simulink model "TRAMI_DCT_AT"  (R2018b)
settings: Solver=FixedStepDiscrete  StartTime=0.0  StopTime=88  FixedStep=10e-3  RelTol=1e-3  EnableMultiTasking=on
undefined symbols (not defined in the file): CONST_AP_GEAR_SUB_NEWTRAL, CONST_AP_IDLE_SPEED_CONT, CONST_AP_LOAD_SFT, CONST_AP_LOAD_SFT_HYS, CONST_CAR_WEIGHT, CONST_CL_NUM, CONST_F_DOWN_SYNCHRO, CONST_F_SYNCHRO, CONST_F_UP_SYNCHRO, CONST_FGR, CONST_I_FlYWHEEL, CONST_INATIA_CLANK, CONST_R_SHIFT_END_CD, CONST_R_SHIFT_END_EG, CONST_R_SHIFT_END_TD, CONST_R_SHIFT_END_UP, CONST_R_SYNCHRO_ENGAGE, CONST_R_TIRE, CONST_RATIO_TQ_REDUCTION, CONST_SKIP_SHIFT_MAX, CONST_SYN_NUM, CONST_T_SFT_END_EN, CONST_T_SFT_END_JUDGE, CONST_T_SFT_END_MAX, CONST_T_SFT_END_MIN, CONST_T_SHIFT_WAIT, CONST_T_TQ_PHASE_CD, CONST_T_TQ_PHASE_ND, CONST_T_TQ_PHASE_NR, CONST_T_TQ_PHASE_TD, CONST_T_TQ_PHASE_UP, CONST_TQ_CREEP_CONT, CONST_TQ_ENGAGE_CL_MARGIN, CONST_TQ_ENGAGE_CL_MIN, CONST_TQ_INATIA_TD_SHIFT, CONST_TQ_LOAD_SFT, CONST_TQ_LOAD_SFT_HYS, CONST_TQ_ND_ENGAGE, CONST_TQ_NR_ENGAGE, CONST_TQ_TQPHASE_MIN, CONST_V_IDLE_SPEED_CONT, Eng, FALSE, GrNP, GrRev, LoopTime, MAT_CL_ENGAGE, MAT_CL_SHARE_RATE, MAT_I_ACTUATOR, MAT_SYNCHRO_COM, MAT_T_GEAR_SUB_NEWTRAL, MAT_TRANS_MGR, MaxCL, Nm, PI, Shift_CD, Shift_ND, Shift_NR, Shift_TD, Shift_Up ... (+168)
libraries: simulink x26
(part 6 of 6)

== system TRAMI_DCT_AT/TCU_Main/StartingDeviceControl/StartingDeviceControl/TCU_Slip_Control/Table_search_3D_G10 ==
  X : Inport  OutDataTypeStr=single
  Y : Inport  Port=2  OutDataTypeStr=single
  1-D Lookup Table1 : Lookup_n-D  NumberOfTableDimensions=1  BreakpointsForDimension1=axis_x  Table=tbl_x  ExtrapMethod=Clip  InternalRulePriority=Speed  OutDataTypeStr=single  RndMeth=Simplest  InputSameDT=on
  1-D Lookup Table2 : Lookup_n-D  NumberOfTableDimensions=1  BreakpointsForDimension1=axis_y  Table=tbl_y  ExtrapMethod=Clip  InternalRulePriority=Speed  OutDataTypeStr=single  RndMeth=Simplest  InputSameDT=on
  2-D Lookup Table : Lookup_n-D  BreakpointsForDimension1=tbl_y  BreakpointsForDimension2=tbl_x  Table=map  ExtrapMethod=Clip  InternalRulePriority=Speed  OutDataTypeStr=single  RndMeth=Simplest  InputSameDT=on
  out : Outport  OutDataTypeStr=single
  wires:
  1-D Lookup Table1/1 -> 2-D Lookup Table/2  "x_nrm"
  1-D Lookup Table2/1 -> 2-D Lookup Table/1  "y_nrm"
  Y/1 -> 1-D Lookup Table2/1  "data_y"
  X/1 -> 1-D Lookup Table1/1  "data_x"
  2-D Lookup Table/1 -> out/1

== system TRAMI_DCT_AT/TCU_Main/StartingDeviceControl/StartingDeviceControl/TCU_Slip_Control/Table_search_3D_G2 ==
  X : Inport  OutDataTypeStr=single
  Y : Inport  Port=2  OutDataTypeStr=single
  1-D Lookup Table1 : Lookup_n-D  NumberOfTableDimensions=1  BreakpointsForDimension1=axis_x  Table=tbl_x  ExtrapMethod=Clip  InternalRulePriority=Speed  OutDataTypeStr=single  RndMeth=Simplest  InputSameDT=on
  1-D Lookup Table2 : Lookup_n-D  NumberOfTableDimensions=1  BreakpointsForDimension1=axis_y  Table=tbl_y  ExtrapMethod=Clip  InternalRulePriority=Speed  OutDataTypeStr=single  RndMeth=Simplest  InputSameDT=on
  2-D Lookup Table : Lookup_n-D  BreakpointsForDimension1=tbl_y  BreakpointsForDimension2=tbl_x  Table=map  ExtrapMethod=Clip  InternalRulePriority=Speed  OutDataTypeStr=single  RndMeth=Simplest  InputSameDT=on
  out : Outport  OutDataTypeStr=single
  wires:
  1-D Lookup Table1/1 -> 2-D Lookup Table/2  "x_nrm"
  1-D Lookup Table2/1 -> 2-D Lookup Table/1  "y_nrm"
  Y/1 -> 1-D Lookup Table2/1  "data_y"
  X/1 -> 1-D Lookup Table1/1  "data_x"
  2-D Lookup Table/1 -> out/1

== system TRAMI_DCT_AT/TCU_Main/StartingDeviceControl/StartingDeviceControl/TCU_Slip_Control/Table_search_3D_G3 ==
  X : Inport  OutDataTypeStr=single
  Y : Inport  Port=2  OutDataTypeStr=single
  1-D Lookup Table1 : Lookup_n-D  NumberOfTableDimensions=1  BreakpointsForDimension1=axis_x  Table=tbl_x  ExtrapMethod=Clip  InternalRulePriority=Speed  OutDataTypeStr=single  RndMeth=Simplest  InputSameDT=on
  1-D Lookup Table2 : Lookup_n-D  NumberOfTableDimensions=1  BreakpointsForDimension1=axis_y  Table=tbl_y  ExtrapMethod=Clip  InternalRulePriority=Speed  OutDataTypeStr=single  RndMeth=Simplest  InputSameDT=on
  2-D Lookup Table : Lookup_n-D  BreakpointsForDimension1=tbl_y  BreakpointsForDimension2=tbl_x  Table=map  ExtrapMethod=Clip  InternalRulePriority=Speed  OutDataTypeStr=single  RndMeth=Simplest  InputSameDT=on
  out : Outport  OutDataTypeStr=single
  wires:
  2-D Lookup Table/1 -> out/1
  X/1 -> 1-D Lookup Table1/1  "data_x"
  Y/1 -> 1-D Lookup Table2/1  "data_y"
  1-D Lookup Table2/1 -> 2-D Lookup Table/1  "y_nrm"
  1-D Lookup Table1/1 -> 2-D Lookup Table/2  "x_nrm"

== system TRAMI_DCT_AT/TCU_Main/StartingDeviceControl/StartingDeviceControl/TCU_Slip_Control/Table_search_3D_G4 ==
  X : Inport  OutDataTypeStr=single
  Y : Inport  Port=2  OutDataTypeStr=single
  1-D Lookup Table1 : Lookup_n-D  NumberOfTableDimensions=1  BreakpointsForDimension1=axis_x  Table=tbl_x  ExtrapMethod=Clip  InternalRulePriority=Speed  OutDataTypeStr=single  RndMeth=Simplest  InputSameDT=on
  1-D Lookup Table2 : Lookup_n-D  NumberOfTableDimensions=1  BreakpointsForDimension1=axis_y  Table=tbl_y  ExtrapMethod=Clip  InternalRulePriority=Speed  OutDataTypeStr=single  RndMeth=Simplest  InputSameDT=on
  2-D Lookup Table : Lookup_n-D  BreakpointsForDimension1=tbl_y  BreakpointsForDimension2=tbl_x  Table=map  ExtrapMethod=Clip  InternalRulePriority=Speed  OutDataTypeStr=single  RndMeth=Simplest  InputSameDT=on
  out : Outport  OutDataTypeStr=single
  wires:
  1-D Lookup Table1/1 -> 2-D Lookup Table/2  "x_nrm"
  1-D Lookup Table2/1 -> 2-D Lookup Table/1  "y_nrm"
  Y/1 -> 1-D Lookup Table2/1  "data_y"
  X/1 -> 1-D Lookup Table1/1  "data_x"
  2-D Lookup Table/1 -> out/1

== system TRAMI_DCT_AT/TCU_Main/StartingDeviceControl/StartingDeviceControl/TCU_Slip_Control/Table_search_3D_G5 ==
  X : Inport  OutDataTypeStr=single
  Y : Inport  Port=2  OutDataTypeStr=single
  1-D Lookup Table1 : Lookup_n-D  NumberOfTableDimensions=1  BreakpointsForDimension1=axis_x  Table=tbl_x  ExtrapMethod=Clip  InternalRulePriority=Speed  OutDataTypeStr=single  RndMeth=Simplest  InputSameDT=on
  1-D Lookup Table2 : Lookup_n-D  NumberOfTableDimensions=1  BreakpointsForDimension1=axis_y  Table=tbl_y  ExtrapMethod=Clip  InternalRulePriority=Speed  OutDataTypeStr=single  RndMeth=Simplest  InputSameDT=on
  2-D Lookup Table : Lookup_n-D  BreakpointsForDimension1=tbl_y  BreakpointsForDimension2=tbl_x  Table=map  ExtrapMethod=Clip  InternalRulePriority=Speed  OutDataTypeStr=single  RndMeth=Simplest  InputSameDT=on
  out : Outport  OutDataTypeStr=single
  wires:
  2-D Lookup Table/1 -> out/1
  X/1 -> 1-D Lookup Table1/1  "data_x"
  Y/1 -> 1-D Lookup Table2/1  "data_y"
  1-D Lookup Table2/1 -> 2-D Lookup Table/1  "y_nrm"
  1-D Lookup Table1/1 -> 2-D Lookup Table/2  "x_nrm"

== system TRAMI_DCT_AT/TCU_Main/StartingDeviceControl/StartingDeviceControl/TCU_Slip_Control/Table_search_3D_G6 ==
  X : Inport  OutDataTypeStr=single
  Y : Inport  Port=2  OutDataTypeStr=single
  1-D Lookup Table1 : Lookup_n-D  NumberOfTableDimensions=1  BreakpointsForDimension1=axis_x  Table=tbl_x  ExtrapMethod=Clip  InternalRulePriority=Speed  OutDataTypeStr=single  RndMeth=Simplest  InputSameDT=on
  1-D Lookup Table2 : Lookup_n-D  NumberOfTableDimensions=1  BreakpointsForDimension1=axis_y  Table=tbl_y  ExtrapMethod=Clip  InternalRulePriority=Speed  OutDataTypeStr=single  RndMeth=Simplest  InputSameDT=on
  2-D Lookup Table : Lookup_n-D  BreakpointsForDimension1=tbl_y  BreakpointsForDimension2=tbl_x  Table=map  ExtrapMethod=Clip  InternalRulePriority=Speed  OutDataTypeStr=single  RndMeth=Simplest  InputSameDT=on
  out : Outport  OutDataTypeStr=single
  wires:
  1-D Lookup Table1/1 -> 2-D Lookup Table/2  "x_nrm"
  1-D Lookup Table2/1 -> 2-D Lookup Table/1  "y_nrm"
  Y/1 -> 1-D Lookup Table2/1  "data_y"
  X/1 -> 1-D Lookup Table1/1  "data_x"
  2-D Lookup Table/1 -> out/1

== system TRAMI_DCT_AT/TCU_Main/StartingDeviceControl/StartingDeviceControl/TCU_Slip_Control/Table_search_3D_G7 ==
  X : Inport  OutDataTypeStr=single
  Y : Inport  Port=2  OutDataTypeStr=single
  1-D Lookup Table1 : Lookup_n-D  NumberOfTableDimensions=1  BreakpointsForDimension1=axis_x  Table=tbl_x  ExtrapMethod=Clip  InternalRulePriority=Speed  OutDataTypeStr=single  RndMeth=Simplest  InputSameDT=on
  1-D Lookup Table2 : Lookup_n-D  NumberOfTableDimensions=1  BreakpointsForDimension1=axis_y  Table=tbl_y  ExtrapMethod=Clip  InternalRulePriority=Speed  OutDataTypeStr=single  RndMeth=Simplest  InputSameDT=on
  2-D Lookup Table : Lookup_n-D  BreakpointsForDimension1=tbl_y  BreakpointsForDimension2=tbl_x  Table=map  ExtrapMethod=Clip  InternalRulePriority=Speed  OutDataTypeStr=single  RndMeth=Simplest  InputSameDT=on
  out : Outport  OutDataTypeStr=single
  wires:
  2-D Lookup Table/1 -> out/1
  X/1 -> 1-D Lookup Table1/1  "data_x"
  Y/1 -> 1-D Lookup Table2/1  "data_y"
  1-D Lookup Table2/1 -> 2-D Lookup Table/1  "y_nrm"
  1-D Lookup Table1/1 -> 2-D Lookup Table/2  "x_nrm"

== system TRAMI_DCT_AT/TCU_Main/StartingDeviceControl/StartingDeviceControl/TCU_Slip_Control/Table_search_3D_G8 ==
  X : Inport  OutDataTypeStr=single
  Y : Inport  Port=2  OutDataTypeStr=single
  1-D Lookup Table1 : Lookup_n-D  NumberOfTableDimensions=1  BreakpointsForDimension1=axis_x  Table=tbl_x  ExtrapMethod=Clip  InternalRulePriority=Speed  OutDataTypeStr=single  RndMeth=Simplest  InputSameDT=on
  1-D Lookup Table2 : Lookup_n-D  NumberOfTableDimensions=1  BreakpointsForDimension1=axis_y  Table=tbl_y  ExtrapMethod=Clip  InternalRulePriority=Speed  OutDataTypeStr=single  RndMeth=Simplest  InputSameDT=on
  2-D Lookup Table : Lookup_n-D  BreakpointsForDimension1=tbl_y  BreakpointsForDimension2=tbl_x  Table=map  ExtrapMethod=Clip  InternalRulePriority=Speed  OutDataTypeStr=single  RndMeth=Simplest  InputSameDT=on
  out : Outport  OutDataTypeStr=single
  wires:
  1-D Lookup Table1/1 -> 2-D Lookup Table/2  "x_nrm"
  1-D Lookup Table2/1 -> 2-D Lookup Table/1  "y_nrm"
  Y/1 -> 1-D Lookup Table2/1  "data_y"
  X/1 -> 1-D Lookup Table1/1  "data_x"
  2-D Lookup Table/1 -> out/1

== system TRAMI_DCT_AT/TCU_Main/StartingDeviceControl/StartingDeviceControl/TCU_Slip_Control/Table_search_3D_G9 ==
  X : Inport  OutDataTypeStr=single
  Y : Inport  Port=2  OutDataTypeStr=single
  1-D Lookup Table1 : Lookup_n-D  NumberOfTableDimensions=1  BreakpointsForDimension1=axis_x  Table=tbl_x  ExtrapMethod=Clip  InternalRulePriority=Speed  OutDataTypeStr=single  RndMeth=Simplest  InputSameDT=on
  1-D Lookup Table2 : Lookup_n-D  NumberOfTableDimensions=1  BreakpointsForDimension1=axis_y  Table=tbl_y  ExtrapMethod=Clip  InternalRulePriority=Speed  OutDataTypeStr=single  RndMeth=Simplest  InputSameDT=on
  2-D Lookup Table : Lookup_n-D  BreakpointsForDimension1=tbl_y  BreakpointsForDimension2=tbl_x  Table=map  ExtrapMethod=Clip  InternalRulePriority=Speed  OutDataTypeStr=single  RndMeth=Simplest  InputSameDT=on
  out : Outport  OutDataTypeStr=single
  wires:
  2-D Lookup Table/1 -> out/1
  X/1 -> 1-D Lookup Table1/1  "data_x"
  Y/1 -> 1-D Lookup Table2/1  "data_y"
  1-D Lookup Table2/1 -> 2-D Lookup Table/1  "y_nrm"
  1-D Lookup Table1/1 -> 2-D Lookup Table/2  "x_nrm"

== system TRAMI_DCT_AT/TCU_Main/StartingDeviceControl/StartingDeviceControl/TCU_Slip_Control/cUnitDelay1 ==
  <param> : Inport
  Constant13 : Constant  Value=initParam  OutDataTypeStr=single
  Switch12 : Switch  Criteria=u2 > Threshold
  Unit Delay2 : UnitDelay  InitialCondition=zeros(size(initParam))  SampleTime=-1
  preParam : Outport
  wires:
  <param>/1 -> Unit Delay2/1
  Constant13/1 -> Switch12/1
  [FlagInit] -> Switch12/2
  Switch12/1 -> preParam/1
  Unit Delay2/1 -> Switch12/3

== system TRAMI_DCT_AT/TCU_Main/StartingDeviceControl/StartingDeviceControl/TCU_Slip_Control/cUnitDelay2 ==
  <param> : Inport
  Constant13 : Constant  Value=initParam  OutDataTypeStr=single
  Switch12 : Switch  Criteria=u2 > Threshold
  Unit Delay2 : UnitDelay  InitialCondition=zeros(size(initParam))  SampleTime=-1
  preParam : Outport
  wires:
  Unit Delay2/1 -> Switch12/3
  Switch12/1 -> preParam/1
  [FlagInit] -> Switch12/2
  Constant13/1 -> Switch12/1
  <param>/1 -> Unit Delay2/1

== system TRAMI_DCT_AT/TCU_Main/ShiftScheduleControl/ShiftScheduleControl/TCU_Gear_Target/calc_gear_target/for_Outer_loop ==
  j : Inport  OutDataTypeStr=int16
  gear_before_shift : Inport  Port=2  OutDataTypeStr=int16
  NUM_LOOP : Inport  Port=3  OutDataTypeStr=int16
  Add : Sum  OutDataTypeStr=int16
  Compare To Constant : simulink/Logic and Bit Operations/Compare To Constant  relop===  const=1  OutDataTypeStr=boolean
  Compare To Constant1 : simulink/Logic and Bit Operations/Compare To Constant  relop===  const=1  OutDataTypeStr=boolean
  Compare To Constant2 : simulink/Logic and Bit Operations/Compare To Constant  relop===  const=-1  OutDataTypeStr=boolean
  Compare To Constant3 : simulink/Logic and Bit Operations/Compare To Constant  relop===  const=-1  OutDataTypeStr=boolean
  For Iterator : ForIterator  ResetStates=reset  IterationSource=external  IndexMode=Zero-based  IterationVariableDataType=int16
  Logical Operator : Logic  AllPortsSameDT=off  OutDataTypeStr=boolean
  Logical Operator1 : Logic  AllPortsSameDT=off  OutDataTypeStr=boolean
  Switch : Switch  Criteria=u2 > Threshold  OutDataTypeStr=int16
  Switch1 : Switch  Criteria=u2 > Threshold  OutDataTypeStr=int16
  Unit Delay : UnitDelay  InitialCondition=-1  SampleTime=-1
  for_inner_loop : Subsystem  TreatAsAtomicUnit=on
  gear_target : Outport  OutDataTypeStr=int16
  wires:
  Switch1/1 -> gear_target/1
  Compare To Constant3/1 -> Switch1/2
  j/1 -> Switch1/1, Add/2
  For Iterator/1 -> Add/1
  NUM_LOOP/1 -> For Iterator/1
  Compare To Constant1/1 -> Logical Operator/2
  for_inner_loop/1(engage_clutch_num) -> Compare To Constant/1
  Compare To Constant/1 -> Logical Operator/1
  for_inner_loop/2(release_clutch_num) -> Compare To Constant1/1
  Logical Operator1/1 -> Switch/2
  Logical Operator/1 -> Logical Operator1/1
  Compare To Constant2/1 -> Logical Operator1/2
  Unit Delay/1 -> Switch/3, Compare To Constant2/1
  Switch/1 -> Compare To Constant3/1, Unit Delay/1, Switch1/3
  gear_before_shift/1 -> for_inner_loop/2(gear_before_shift)
  Add/1 -> Switch/1, for_inner_loop/1(j)

== system TRAMI_DCT_AT/TCU_Main/ShiftScheduleControl/ShiftScheduleControl/TCU_Gear_Target/calc_gear_target/for_Outer_loop/for_inner_loop ==
  j : Inport  OutDataTypeStr=int16
  gear_before_shift : Inport  Port=2  OutDataTypeStr=int16
  Add2 : Sum  Inputs=+  OutDataTypeStr=int16
  Add3 : Sum  Inputs=+  OutDataTypeStr=int16
  Compare To Constant : simulink/Logic and Bit Operations/Compare To Constant  relop===  const=0  OutDataTypeStr=boolean
  Compare To Constant1 : simulink/Logic and Bit Operations/Compare To Constant  relop=>  const=0  OutDataTypeStr=boolean
  Compare To Constant2 : simulink/Logic and Bit Operations/Compare To Constant  relop=>  const=0  OutDataTypeStr=boolean
  Compare To Constant3 : simulink/Logic and Bit Operations/Compare To Constant  relop===  const=0  OutDataTypeStr=boolean
  Constant : Constant  Value=[0:MaxCL-1]  OutDataTypeStr=single
  Data Type Conversion : DataTypeConversion  OutDataTypeStr=int16
  Data Type Conversion1 : DataTypeConversion  OutDataTypeStr=int16
  Direct Lookup Table (n-D) : LookupNDDirect  Table=MAT_CL_ENGAGE
  Direct Lookup Table (n-D)1 : LookupNDDirect  Table=MAT_CL_ENGAGE
  Logical Operator : Logic  AllPortsSameDT=off  OutDataTypeStr=boolean
  Logical Operator1 : Logic  AllPortsSameDT=off  OutDataTypeStr=boolean
  engage_clutch_num : Outport  OutDataTypeStr=int16
  release_clutch_num : Outport  Port=2  OutDataTypeStr=int16
  wires:
  Data Type Conversion1/1 -> Add3/1
  Data Type Conversion/1 -> Add2/1
  Logical Operator1/1 -> Data Type Conversion1/1
  Logical Operator/1 -> Data Type Conversion/1
  Add3/1 -> release_clutch_num/1
  Add2/1 -> engage_clutch_num/1
  Compare To Constant3/1 -> Logical Operator1/2
  Compare To Constant2/1 -> Logical Operator1/1
  j/1 -> Direct Lookup Table (n-D)1/2
  Constant/1 -> Direct Lookup Table (n-D)/1, Direct Lookup Table (n-D)1/1
  Compare To Constant/1 -> Logical Operator/1
  Direct Lookup Table (n-D)1/1 -> Compare To Constant1/1, Compare To Constant3/1
  Compare To Constant1/1 -> Logical Operator/2
  Direct Lookup Table (n-D)/1 -> Compare To Constant/1, Compare To Constant2/1
  gear_before_shift/1 -> Direct Lookup Table (n-D)/2
